simulink model "spring_damper"  (R2019b)
settings: Solver=VariableStepAuto  StartTime=0.0  StopTime=sim_time  MaxStep=0.01  RelTol=1e-3
values from neighbouring files (symbols this model uses):
  b = 50    [adaptive_cruise.m]    (also in damper_pid_run.m = 10; dc_motor_run.m = 3.5077e-06; pid_tune_run.m = 10; spring_damp.m = 0.5)
  F = 2    [diff_int.m]    (also in spring_damp.m = 1)
  k = 20    [damper_pid_run.m]    (also in pid_tune_run.m; spring_damp.m)
  M = 1    [damper_pid_run.m]    (also in pid_tune_run.m; spring_damp.m)
libraries: dspsrcs4 x1
settings Model: Creator=dgander  LastModifiedBy=dgander

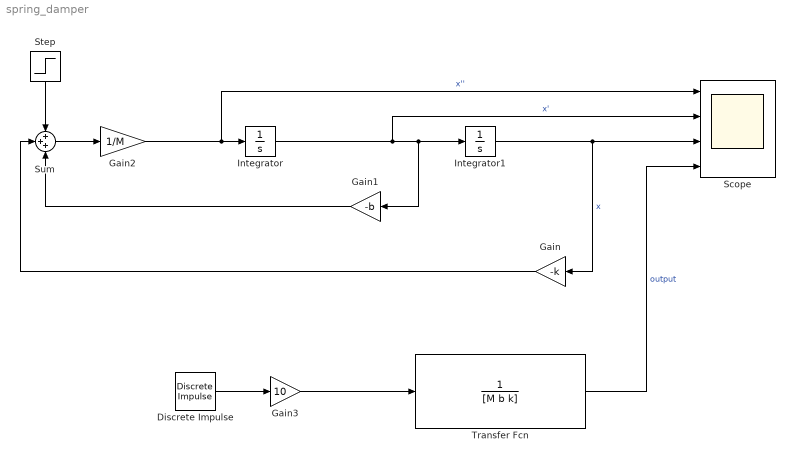
== system spring_damper ==
  Discrete Impulse : dspsrcs4/Discrete  Impulse  Delay=0  SampleTime=1  FrameSample=1  OutputFrames=off  dataType=double  isSigned=on  wordLen=16  udDataType=sfix(16)  fracBitsMode=Best precision  numFracBits=15  OutDataTypeStr=double  LastOutDataTypeStr=double
  Gain : Gain  Gain=-k
  Gain1 : Gain  Gain=-b
  Gain2 : Gain  Gain=1/M
  Gain3 : Gain  Gain=10
  Integrator : Integrator
  Integrator1 : Integrator
  Scope : Scope  NumInputPorts=4
  Step : Step  After=F  SampleTime=0
  Sum : Sum  Inputs=+++
  Transfer Fcn : TransferFcn  Denominator=[M b k]
  wires:
  Gain2/1 -> Scope/1, Integrator/1  "x''"
  Integrator/1 -> Scope/2, Gain1/1, Integrator1/1  "x'"
  Integrator1/1 -> Gain/1, Scope/3  "x"
  Gain1/1 -> Sum/3
  Step/1 -> Sum/1
  Gain/1 -> Sum/2
  Sum/1 -> Gain2/1
  Transfer Fcn/1 -> Scope/4  "output"
  Discrete Impulse/1 -> Gain3/1
  Gain3/1 -> Transfer Fcn/1
